simulink model "MSICA_Projet1_StructureModaleObservateur"  (R2018a)
settings: Solver=VariableStepAuto  StartTime=0.0  StopTime=10.0  RelTol=1e-3
values from neighbouring files (symbols this model uses):
  Amod = [zeros(3) eye(3); -omega_carre -2*xi*sqrt(omega_carre)]    [DonneesProjet.m]
  Bmod = [zeros(3); phi']    [DonneesProjet.m]
  Cmod = [phi zeros(3,3)]    [DonneesProjet.m]
libraries: Blocs_LTI x2
settings Model: Creator=natha  LastModifiedBy=natha
settings DataIOCC: ReturnWorkspaceOutputs=on
settings SFSimCC: SimUseLocalCustomCode=on
settings RTWCC: RTWUseLocalCustomCode=on

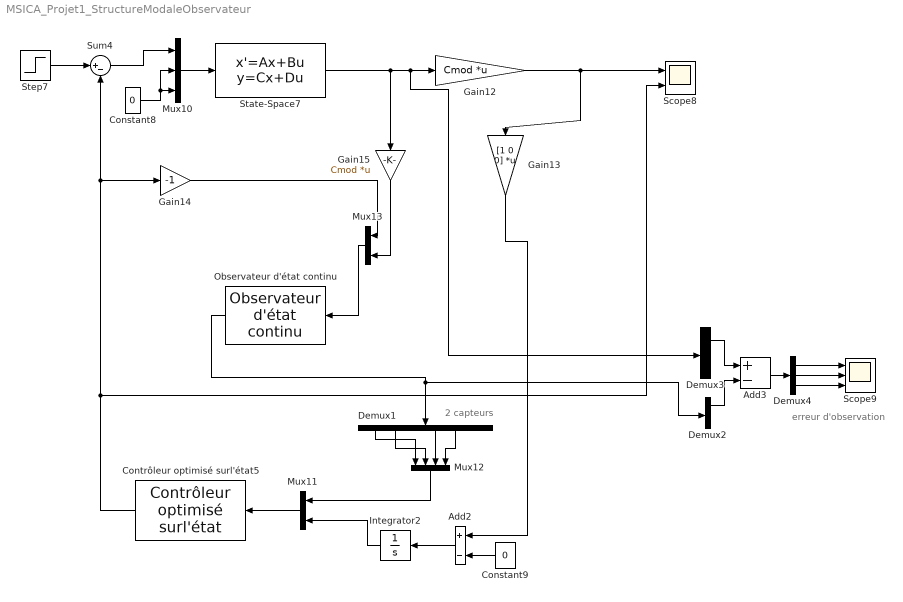
== system MSICA_Projet1_StructureModaleObservateur ==
  note: erreur d'observation
  note: 2 capteurs
  Add2 : Sum  Inputs=+-
  Add3 : Sum  Inputs=+-
  Constant8 : Constant  Value=0
  Constant9 : Constant  Value=0
  Contrôleur optimisé surl'état5 : Blocs_LTI/Contrôleur optimisé surl'état  MaskParameter1=Amod2cont  MaskParameter2=Bcont  MaskParameter3=diag([1e3 1e3 1e5 1e5 1e13])  MaskParameter4=eye(1,1)
  Demux1 : Demux  Outputs=6
  Demux2 : Demux  Outputs=2
  Demux3 : Demux  Outputs=2
  Demux4 : Demux  Outputs=3
  Gain12 : Gain  Gain=Cmod  Multiplication=Matrix(K*u)
  Gain13 : Gain  Gain=[1 0 0]  Multiplication=Matrix(K*u)
  Gain14 : Gain  Gain=-1
  Gain15 : Gain  Gain=Cmod  Multiplication=Matrix(K*u)
  Integrator2 : Integrator
  Mux10 : Mux  Inputs=3
  Mux11 : Mux  Inputs=2
  Mux12 : Mux
  Mux13 : Mux  Inputs=2
  Observateur d'état continu : Blocs_LTI/Observateur d'état continu  MaskParameter1=Amod  MaskParameter2=Bmod(:,1)  MaskParameter3=[phi zeros(3)]  MaskParameter4=zeros(3,1)  MaskParameter5=0.001*Bmod(:,1)*Bmod(:,1)'  MaskParameter6=0.01*eye(3)
  Scope8 : Scope  NumInputPorts=2
  Scope9 : Scope  NumInputPorts=3
  State-Space7 : StateSpace  A=Amod  B=Bmod  C=eye(6)  D=zeros(6,3)  InitialCondition=0
  Step7 : Step  Time=0  After=10  SampleTime=0
  Sum4 : Sum  Inputs=|+-
  wires:
  Integrator2/1 -> Mux11/2
  Gain14/1 -> Mux13/1
  Demux1/5 -> Mux12/4
  Add3/1 -> Demux4/1
  Mux12/1 -> Mux11/1
  Constant8/1 -> Mux10/2, Mux10/3
  Contrôleur optimisé surl'état5/1 -> Gain14/1, Sum4/2, Scope8/2
  Add2/1 -> Integrator2/1
  State-Space7/1 -> Demux3/1, Gain12/1, Gain15/1
  Mux11/1 -> Contrôleur optimisé surl'état5/1
  Demux4/1 -> Scope9/1
  Demux1/4 -> Mux12/3
  Gain12/1 -> Scope8/1, Gain13/1
  Gain15/1 -> Mux13/2
  Mux10/1 -> State-Space7/1
  Gain13/1 -> Add2/1
  Sum4/1 -> Mux10/1
  Demux4/2 -> Scope9/2
  Demux1/1 -> Mux12/1
  Demux4/3 -> Scope9/3
  Constant9/1 -> Add2/2
  Observateur d'état continu/1 -> Demux2/1, Demux1/1
  Demux2/1 -> Add3/2
  Step7/1 -> Sum4/1
  Demux1/2 -> Mux12/2
  Mux13/1 -> Observateur d'état continu/1
  Demux3/1 -> Add3/1
